simulink model "Examp_algebra1"  (R2014a)
settings: Solver=ode3  StartTime=0.0  StopTime=5.0  FixedStep=0.01  RelTol=1e-3
libraries: simulink x1
settings Model: Creator=Administrator  LastModifiedBy=李广文
settings DataIOCC: SignalLoggingSaveFormat=ModelDataLogs  SignalLoggingName=sigsOut
settings OptimizationCC: ExpressionDepthLimit=2147483647  InitFltsAndDblsToZero=on
settings DebuggingCC: SaveWithParameterizedLinksMsg=none  UnderspecifiedInitializationDetection=Classic  SignalResolutionControl=TryResolveAllWithWarning  SolverPrmCheckMsg=none  MultiTaskDSMMsg=warning  MultiTaskCondExecSysMsg=none  FcnCallInpInsideContextMsg=UseLocalSettings  StateNameClashWarn=warning
settings HardwareCC: TargetUnknown=on
settings RTWCC: IncludeERTFirstTime=on
settings GRTTargetCC: TargetFcnLib=ansi_tfl_tmw.mat  CombineOutputUpdateFcns=off  GRTInterface=on

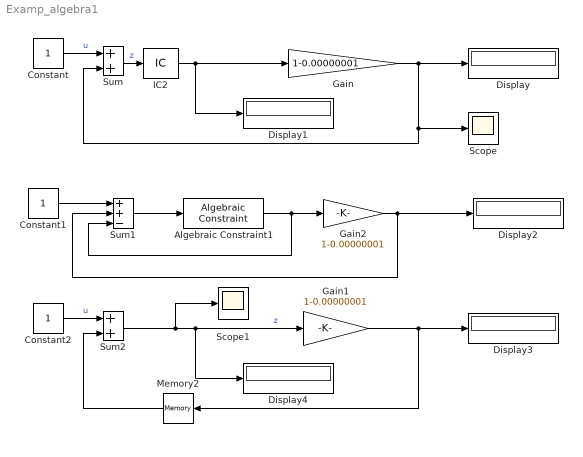
== system Examp_algebra1 ==
  Algebraic Constraint1 : simulink/Math Operations/Algebraic Constraint  z0=10
  Constant : Constant
  Constant1 : Constant
  Constant2 : Constant
  Display{,1..4} (5 alike) : Display
  Gain : Gain  Gain=1-0.00000001
  Gain1 : Gain  Gain=1-0.00000001
  Gain2 : Gain  Gain=1-0.00000001
  IC2 : InitialCondition  Value=100
  Memory2 : Memory
  Scope : Scope
  Scope1 : Scope
  Sum : Sum  SaturateOnIntegerOverflow=on
  Sum1 : Sum  Inputs=++-  SaturateOnIntegerOverflow=on
  Sum2 : Sum  SaturateOnIntegerOverflow=on
  wires:
  Gain/1 -> Sum/2, Scope/1, Display/1
  Sum/1 -> IC2/1  "z"
  Constant/1 -> Sum/1  "u"
  Constant1/1 -> Sum1/1
  Sum1/1 -> Algebraic Constraint1/1
  Algebraic Constraint1/1 -> Sum1/3, Gain2/1
  Gain2/1 -> Display2/1, Sum1/2
  Gain1/1 -> Memory2/1, Display3/1
  Sum2/1 -> Scope1/1, Display4/1, Gain1/1  "z"
  Constant2/1 -> Sum2/1  "u"
  Memory2/1 -> Sum2/2
  IC2/1 -> Gain/1, Display1/1
